simulink model "sedemo_nd_attributes"  (Simulink 7.5)
settings: Solver=VariableStepDiscrete  StartTime=0.0  StopTime=1  MaxStep=inf  RelTol=1e-3
PreLoadFcn:
  | image_source=imread('sedemo_onion.png');
  | imghdl=[];
StopFcn:
  | try
  |     imghdl=imageview(uint8(image_dest.signals.values(:,:,:,end)));
  | end
  | try
  |     set(imghdl,'Name','Received Image');
  | end
libraries: simeventssink1 x2, simeventsgenerators1 x2, simeventsattributes2 x2, simeventsserver1 x1, simeventsinfo x1
CloseFcn:
  | try
  |     close(imghdl);
  | end
  | try
  |     clear image_source image_dest imghdl;
  | end
settings Model: Creator=The MathWorks Inc.  ExtModeAutoUpdateStatusClock=off
settings DataIOCC: SaveOutput=off  SaveTime=off
settings OptimizationCC: InitFltsAndDblsToZero=on
settings DebuggingCC: AlgebraicLoopMsg=error  SignalResolutionControl=TryResolveAllWithWarning  SolverPrmCheckMsg=none  StrictBusMsg=Warning
settings SimEventsCC: propDiagAttribOutput=1  propDiagFcnCallOutput=1  propDiagStatOutput=0

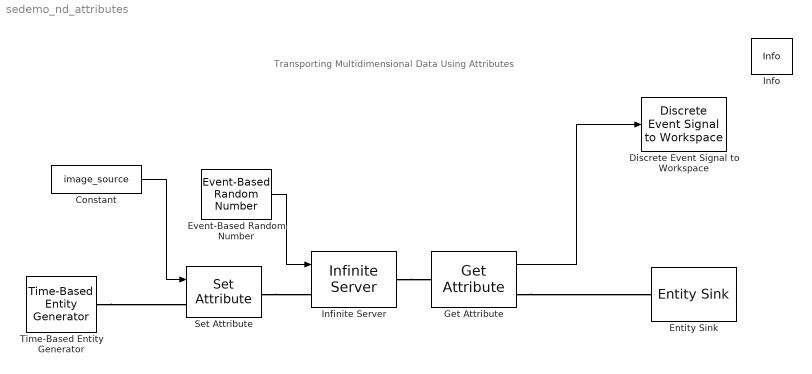
== system sedemo_nd_attributes ==
  note: Transporting Multidimensional Data Using Attributes
  Constant : Constant  Value=image_source  OutDataTypeMode=double  OutDataType=sfix(16)  OutScaling=2^0  OutDataTypeStr=double
  Discrete Event Signal to Workspace : simeventssink1/Discrete Event Signal to Workspace  SystemSampleTime=-1  VariableName=image_dest  SaveFormat=Structure With Time  IsMonitorOnly=off  IsRecordIC=off
  Entity Sink : simeventssink1/Entity Sink  Priority=1  SystemSampleTime=-1  AvailableForArrivals=on  StatNumberArrived=Off
  Event-Based Random Number : simeventsgenerators1/Signal Generators/Event-Based Random Number  SystemSampleTime=-1  distribution=Uniform  meanExp=1  minUnif=0  maxUnif=1  pOneBern=0.25  pSuccessBino=0.5  numTrialBino=1  meanNorm=0  stdNorm=1  minTri=1  maxTri=3  modeTri=2  thresholdLogn=0  scaleLogn=1  shapeLogn=1  pSuccessGeo=0.5  meanPoiss=1  thresholdLogl=0  scaleLogl=1  thresholdGam=0  scaleGam=1  shapeGam=1  minBeta=0  maxBeta=1  shape1Beta=1  shape2Beta=1  minUnid=0  maxUnid=1  numValueUnid=2  thresholdWbl=0  scaleWbl=1  shapeWbl=1  valueVecCont=[0 1]  cdfVecCont=[0 1]  valueVecDisc=[0 1]  probVecDisc=[0.5 0.5]  seed=12345  IsProcessed=on  isConnected=1
  Get Attribute : simeventsattributes2/Get Attribute  Priority=1  DialogController=des_ddg_create  DialogControllerArgs=DataTag2  SystemSampleTime=-1  AttributeName=EntityIndex  AttributeMissing=Error  AttributeDefaultValue=1  AttributeSendTiming=After entity departure  AttributeTreatAsVector=1  StatNumberDeparted=Off  EvaluatedDefaultAttributeValue={[]}
  Infinite Server : simeventsserver1/Infinite Server  Priority=1  SystemSampleTime=-1  ServiceTimeFrom=Signal port t  ServiceTime=1  AttributeName=ServiceTime  PriorityServiceCompletion=500  EnableTOPort=off  StatNumberDeparted=Off  StatNumberInBlock=Off  StatPendingEntity=Off  StatNumberPending=Off  StatAverageWait=Off  StatNumberTimedout=Off
  Info : simeventsinfo/Info  SystemSampleTime=-1
  Set Attribute : simeventsattributes2/Set Attribute  Priority=1  DialogController=des_ddg_create  DialogControllerArgs=DataTag5  SystemSampleTime=-1  AttributeFrom=Signal port  AttributeName=EntityIndex  AttributeTreatAsVector=1  AttributeValue=1  AttributeCreate=on  StatNumberDeparted=Off  EvaluatedAttributeValue={[]}
  Time-Based Entity Generator : simeventsgenerators1/Entity Generators/Time-Based Entity Generator  Priority=1  DialogController=des_ddg_create  DialogControllerArgs=DataTag7  SystemSampleTime=-1  GenerateEntitiesUpon=Intergeneration time from dialog  Distribution=Constant  Minimum=0  Maximum=1  Mean=1  InitialSeed=12345  Period=100  PriorityEntityGeneration=1  GenerateEntityAtSimulationStart=on  ResponseWhenBlocked=Pause generation  ResponseWhenUnblocked=Immediate restart  EntityType=Standard  StatNumberDeparted=Off  StatPendingEntity=Off  StatAverageIntergenerationTime=Off
  wires:
  Event-Based Random Number/1 -> Infinite Server/1
  Constant/1 -> Set Attribute/1
  Get Attribute/1 -> Discrete Event Signal to Workspace/1
  connections:
  Time-Based Entity Generator/RConn1 -- Set Attribute/LConn1
  Set Attribute/RConn1 -- Infinite Server/LConn1
  Infinite Server/RConn1 -- Get Attribute/LConn1
  Get Attribute/RConn1 -- Entity Sink/LConn1
